simulink model "directionController"  (R2016b)
settings: Solver=FixedStepAuto  StartTime=0.0  StopTime=inf  RelTol=1e-3
libraries: robotlib x5
settings Model: Creator=jupan  LastModifiedBy=jupan
settings OptimizationCC: MaxStackSize=64
settings DebuggingCC: ParameterTunabilityLossMsg=error
settings HardwareCC: ProdBitPerPointer=32  ProdBitPerSizeT=32  ProdBitPerPtrDiffT=32  ProdLargestAtomicFloat=None  ProdIntDivRoundTo=Undefined  ProdEndianess=Unspecified  ProdWordSize=32  ProdHWDeviceType=Generic->Unspecified (assume 32-bit Generic)
settings RTWCC: SystemTargetFile=ert.tlc  HardwareBoard=Robot Operating System (ROS)  TLCOptions="-aInlineSetEventsForThisBaseRateFcn=TLC_FALSE -aSuppressMultiTaskScheduler=TLC_FALSE  -aRateBasedStepFcn=0"  TemplateMakefile=ert_default_tmf  Description=Embedded Coder  GenerateReport=on  Toolchain=Catkin  IncludeHyperlinkInReport=on  LaunchReport=on  TargetLang=C++  GenerateTraceInfo=on  GenerateTraceReport=on  GenerateTraceReportSl=on  GenerateTraceReportSf=on  GenerateTraceReportEml=on
settings CodeAppCC: ForceParamTrailComments=on  IgnoreCustomStorageClasses=off  OperatorAnnotations=on  SimulinkDataObjDesc=on  SFDataObjDesc=on  MATLABFcnDesc=on  InsertBlockDesc=on  MATLABSourceComments=on

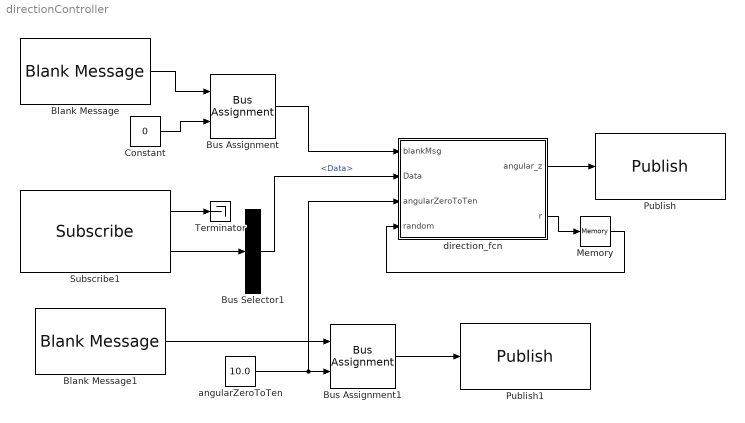
== system directionController ==
  Blank Message : robotlib/Blank Message  SourceLibraryInfo=This block requires Robotics System Toolbox  messageType=std_msgs/Float64  SampleTime=inf
  Blank Message1 : robotlib/Blank Message  SourceLibraryInfo=This block requires Robotics System Toolbox  messageType=std_msgs/Float64  SampleTime=inf
  Bus Assignment : BusAssignment  AssignedSignals=Data
  Bus Assignment1 : BusAssignment  AssignedSignals=Data
  Bus Selector1 : BusSelector  OutputSignals=Data
  Constant : Constant  Value=0
  Memory : Memory
  Publish : robotlib/Publish  SourceLibraryInfo=This block requires Robotics System Toolbox  topicSource=Specify your own  topic=/direction  messageType=std_msgs/Float64  messageQueueLength=1
  Publish1 : robotlib/Publish  SourceLibraryInfo=This block requires Robotics System Toolbox  topicSource=Specify your own  topic=/directionController/angularZeroToTen  messageType=std_msgs/Float64  messageQueueLength=1
  Subscribe1 : robotlib/Subscribe  SourceLibraryInfo=This block requires Robotics System Toolbox  topicSource=Select from ROS network  topic=/catvehicle/distanceEstimator/dist  messageType=std_msgs/Float32  sampleTime=-1  messageQueueLength=1
  Terminator : Terminator
  angularZeroToTen : Constant  Value=10.0  OutDataTypeStr=double
  direction_fcn : MATLAB Function  TreatAsAtomicUnit=on
  wires:
  Subscribe1/2 -> Bus Selector1/1
  Bus Selector1/1 -> direction_fcn/2(Data)  "<Data>"
  Subscribe1/1 -> Terminator/1
  Blank Message/1 -> Bus Assignment/1
  direction_fcn/1(angular_z) -> Publish/1
  Bus Assignment/1 -> direction_fcn/1(blankMsg)
  Constant/1 -> Bus Assignment/2
  Blank Message1/1 -> Bus Assignment1/1
  angularZeroToTen/1 -> direction_fcn/3(angularZeroToTen), Bus Assignment1/2
  Bus Assignment1/1 -> Publish1/1
  direction_fcn/2(r) -> Memory/1
  Memory/1 -> direction_fcn/4(random)

== matlab function directionController/direction_fcn ==
  data: blankMsg input; Data input; angular_z output SL_Bus_directionController_std_msgs_Float64; angularZeroToTen input; random input; r output
function [angular_z, r] = fcn(blankMsg, Data, angularZeroToTen, random)

angular_z = blankMsg;

if(Data > 0 && Data < 10)
    if(random == 0) 
        % Turning left;
        angular_z.Data = angularZeroToTen;
        r = random;
    else
        % Turning right;
        angular_z.Data = -angularZeroToTen;
        r = random;
    end
else
    angular_z.Data = 0;
    r = randi([0 1], 1, 1);
end
